simulink model "pattern_separation"  (R2019b)
settings: Solver=FixedStepAuto  StartTime=1  StopTime=simulationtime  FixedStep=stepsize  RelTol=1e-3
values from neighbouring files (symbols this model uses):
  a1 = 0.02    [simulation.m]
  a2 = 0.02    [simulation.m]
  b1 = 0.025    [simulation.m]
  b2 = 0.04    [simulation.m]
  c1 = -65    [simulation.m]
  C1 = normrnd(100,10,[1,nrofgranulecells])    [simulation.m]
  c2 = -65    [simulation.m]
  C2 = normrnd(100,10,[1,nrofinterneurons])    [simulation.m]
  d1 = 6    [simulation.m]
  d2 = 2    [simulation.m]
  inputset = inputsets{no_input}    [simulation.m]
  k1 = 0.25    [simulation.m]
  k2 = 0.25    [simulation.m]
  minimum_saturation_limit_1 = -80    [simulation.m]
  minimum_saturation_limit_2 = -100    [simulation.m]
  noumberofevents = 500    [simulation.m]
  Re = 230    [simulation.m]
  simulationtime = 2000    [simulation.m]
  stepsize = 1    [simulation.m]
  ve1 = -5    [simulation.m]
  ve2 = -80    [simulation.m]
  vr1 = -60    [simulation.m]
  vr2 = -65    [simulation.m]
  vt1 = -55    [simulation.m]
  vt2 = -48    [simulation.m]
undefined symbols (not defined in the file or in its folder): conductancemaxima1, conductancemaxima2, conductancemaxima3, decaytimes1, decaytimes2, decaytimes3, DiscIntNeverNeededParam, Nd, trace
(part 5 of 5)

== matlab function pattern_separation/granule cell 13/MATLAB Function1 ==
  data: eventnoumber input; decaytime output; decaytimes1 input; conductancemaxima1 input; conductancemaximum output
function [decaytime, conductancemaximum] = fcn(eventnoumber, decaytimes1, conductancemaxima1)
if eventnoumber ==0
decaytime =1;
conductancemaximum =0;
else
decaytime = decaytimes1(13, eventnoumber);
conductancemaximum = conductancemaxima1(13, eventnoumber);
end

== matlab function pattern_separation/granule cell 13/MATLAB Function2 ==
  data: eventnoumber input; decaytime output; decaytimes2 input; conductancemaxima2 input; conductancemaximum output
function [decaytime, conductancemaximum] = fcn(eventnoumber, decaytimes2, conductancemaxima2)
if eventnoumber ==0
decaytime =1;
conductancemaximum =0;
else
decaytime = decaytimes2(13, eventnoumber);
conductancemaximum = conductancemaxima2(13, eventnoumber);
end

== matlab function pattern_separation/granule cell 13/granule cell/reset function ==
  data: v input; c input; d input; u input; v1 output; u1 output; r output

function [v1,u1,r] = fcn(v,c,d,u)

if v >= 30
v1= c;
u1 = u+d;
r=1;
else
v1=v;
u1=u;
r=0;  
end

== matlab function pattern_separation/granule cell 1/MATLAB Function2 ==
  data: eventnoumber input; decaytime output; decaytimes2 input; conductancemaxima2 input; conductancemaximum output
function [decaytime, conductancemaximum] = fcn(eventnoumber, decaytimes2, conductancemaxima2)
if eventnoumber ==0
decaytime =1;
conductancemaximum =0;
else
decaytime = decaytimes2(1, eventnoumber);
conductancemaximum = conductancemaxima2(1, eventnoumber);
end

== matlab function pattern_separation/granule cell 1/single exp IPSCs generator (ihibitory synapse)/MATLAB Function ==
  data: inp input; exponential output
function exponential = fcn(inp)

exponential = exp(-inp);

== matlab function pattern_separation/granule cell 13/single exp EPSCs generator (recurrent synapse)/MATLAB Function ==
  data: inp input; exponential output
function exponential = fcn(inp)

exponential = exp(-inp);

== matlab function pattern_separation/granule cell 13/single exp IPSCs generator (ihibitory synapse)/MATLAB Function ==
  data: inp input; exponential output
function exponential = fcn(inp)

exponential = exp(-inp);

== matlab function pattern_separation/granule cell 14/GC neuron/reset function ==
  data: v input; c input; d input; u input; v1 output; u1 output; r output

function [v1,u1,r] = fcn(v,c,d,u)

if v >= 30
v1= c;
u1 = u+d;
r=1;
else
v1=v;
u1=u;
r=0;  
end

== matlab function pattern_separation/granule cell 14/MATLAB Function1 ==
  data: eventnoumber input; decaytime output; decaytimes1 input; conductancemaxima1 input; conductancemaximum output
function [decaytime, conductancemaximum] = fcn(eventnoumber, decaytimes1, conductancemaxima1)
if eventnoumber ==0
decaytime =1;
conductancemaximum =0;
else
decaytime = decaytimes1(14, eventnoumber);
conductancemaximum = conductancemaxima1(14, eventnoumber);
end

== matlab function pattern_separation/granule cell 1/MATLAB Function1 ==
  data: eventnoumber input; decaytime output; decaytimes1 input; conductancemaxima1 input; conductancemaximum output
function [decaytime, conductancemaximum] = fcn(eventnoumber, decaytimes1, conductancemaxima1)
if eventnoumber ==0
decaytime =1;
conductancemaximum =0;
else
decaytime = decaytimes1(1, eventnoumber);
conductancemaximum = conductancemaxima1(1, eventnoumber);
end

== matlab function pattern_separation/granule cell 1/single exp EPSCs generator (recurrent synapse)/MATLAB Function ==
  data: inp input; exponential output
function exponential = fcn(inp)

exponential = exp(-inp);

== matlab function pattern_separation/granule cell 14/MATLAB Function2 ==
  data: eventnoumber input; decaytime output; decaytimes2 input; conductancemaxima2 input; conductancemaximum output
function [decaytime, conductancemaximum] = fcn(eventnoumber, decaytimes2, conductancemaxima2)
if eventnoumber ==0
decaytime =1;
conductancemaximum =0;
else
decaytime = decaytimes2(14, eventnoumber);
conductancemaximum = conductancemaxima2(14, eventnoumber);
end

== matlab function pattern_separation/granule cell 14/single exp EPSCs generator (recurrent synapse)/MATLAB Function ==
  data: inp input; exponential output
function exponential = fcn(inp)

exponential = exp(-inp);

== matlab function pattern_separation/granule cell 14/single exp IPSCs generator (ihibitory synapse)/MATLAB Function ==
  data: inp input; exponential output
function exponential = fcn(inp)

exponential = exp(-inp);

== matlab function pattern_separation/granule cell 15/MATLAB Function1 ==
  data: eventnoumber input; decaytime output; decaytimes1 input; conductancemaxima1 input; conductancemaximum output
function [decaytime, conductancemaximum] = fcn(eventnoumber, decaytimes1, conductancemaxima1)
if eventnoumber ==0
decaytime =1;
conductancemaximum =0;
else
decaytime = decaytimes1(15, eventnoumber);
conductancemaximum = conductancemaxima1(15, eventnoumber);
end

== matlab function pattern_separation/granule cell 15/MATLAB Function2 ==
  data: eventnoumber input; decaytime output; decaytimes2 input; conductancemaxima2 input; conductancemaximum output
function [decaytime, conductancemaximum] = fcn(eventnoumber, decaytimes2, conductancemaxima2)
if eventnoumber ==0
decaytime =1;
conductancemaximum =0;
else
decaytime = decaytimes2(15, eventnoumber);
conductancemaximum = conductancemaxima2(15, eventnoumber);
end

== matlab function pattern_separation/granule cell 15/granule cell/reset function ==
  data: v input; c input; d input; u input; v1 output; u1 output; r output

function [v1,u1,r] = fcn(v,c,d,u)

if v >= 30
v1= c;
u1 = u+d;
r=1;
else
v1=v;
u1=u;
r=0;  
end

== matlab function pattern_separation/granule cell 15/single exp EPSCs generator (recurrent synapse)/MATLAB Function ==
  data: inp input; exponential output
function exponential = fcn(inp)

exponential = exp(-inp);

== matlab function pattern_separation/granule cell 15/single exp IPSCs generator (ihibitory synapse)/MATLAB Function ==
  data: inp input; exponential output
function exponential = fcn(inp)

exponential = exp(-inp);

== matlab function pattern_separation/granule cell 16/GC neuron/reset function ==
  data: v input; c input; d input; u input; v1 output; u1 output; r output

function [v1,u1,r] = fcn(v,c,d,u)

if v >= 30
v1= c;
u1 = u+d;
r=1;
else
v1=v;
u1=u;
r=0;  
end

== matlab function pattern_separation/granule cell 16/MATLAB Function1 ==
  data: eventnoumber input; decaytime output; decaytimes1 input; conductancemaxima1 input; conductancemaximum output
function [decaytime, conductancemaximum] = fcn(eventnoumber, decaytimes1, conductancemaxima1)
if eventnoumber ==0
decaytime =1;
conductancemaximum =0;
else
decaytime = decaytimes1(16, eventnoumber);
conductancemaximum = conductancemaxima1(16, eventnoumber);
end

== matlab function pattern_separation/granule cell 16/MATLAB Function2 ==
  data: eventnoumber input; decaytime output; decaytimes2 input; conductancemaxima2 input; conductancemaximum output
function [decaytime, conductancemaximum] = fcn(eventnoumber, decaytimes2, conductancemaxima2)
if eventnoumber ==0
decaytime =1;
conductancemaximum =0;
else
decaytime = decaytimes2(16, eventnoumber);
conductancemaximum = conductancemaxima2(16, eventnoumber);
end

== matlab function pattern_separation/granule cell 16/single exp EPSCs generator (recurrent synapse)/MATLAB Function ==
  data: inp input; exponential output
function exponential = fcn(inp)

exponential = exp(-inp);

== matlab function pattern_separation/granule cell 16/single exp IPSCs generator (ihibitory synapse)/MATLAB Function ==
  data: inp input; exponential output
function exponential = fcn(inp)

exponential = exp(-inp);

== matlab function pattern_separation/granule cell 9/MATLAB Function1 ==
  data: eventnoumber input; decaytime output; decaytimes1 input; conductancemaxima1 input; conductancemaximum output
function [decaytime, conductancemaximum] = fcn(eventnoumber, decaytimes1, conductancemaxima1)
if eventnoumber ==0
decaytime =1;
conductancemaximum =0;
else
decaytime = decaytimes1(9, eventnoumber);
conductancemaximum = conductancemaxima1(9, eventnoumber);
end

== matlab function pattern_separation/granule cell 9/MATLAB Function2 ==
  data: eventnoumber input; decaytime output; decaytimes2 input; conductancemaxima2 input; conductancemaximum output
function [decaytime, conductancemaximum] = fcn(eventnoumber, decaytimes2, conductancemaxima2)
if eventnoumber ==0
decaytime =1;
conductancemaximum =0;
else
decaytime = decaytimes2(9, eventnoumber);
conductancemaximum = conductancemaxima2(9, eventnoumber);
end

== matlab function pattern_separation/granule cell 9/granule cell/reset function ==
  data: v input; c input; d input; u input; v1 output; u1 output; r output

function [v1,u1,r] = fcn(v,c,d,u)

if v >= 30
v1= c;
u1 = u+d;
r=1;
else
v1=v;
u1=u;
r=0;  
end

== matlab function pattern_separation/granule cell 9/single exp EPSCs generator (recurrent synapse)/MATLAB Function ==
  data: inp input; exponential output
function exponential = fcn(inp)

exponential = exp(-inp);

== matlab function pattern_separation/granule cell 9/single exp IPSCs generator (ihibitory synapse)/MATLAB Function ==
  data: inp input; exponential output
function exponential = fcn(inp)

exponential = exp(-inp);

== matlab function pattern_separation/stimulation (pattern generator)/MATLAB Function ==
  data: iteration input; integrator input; trigger output; spiketrains input
function trigger = fcn(iteration, integrator,spiketrains)
trigger = spiketrains(iteration,integrator);

== matlab function pattern_separation/granule cell 17/MATLAB Function1 ==
  data: eventnoumber input; decaytime output; decaytimes1 input; conductancemaxima1 input; conductancemaximum output
function [decaytime, conductancemaximum] = fcn(eventnoumber, decaytimes1, conductancemaxima1)
if eventnoumber ==0
decaytime =1;
conductancemaximum =0;
else
decaytime = decaytimes1(17, eventnoumber);
conductancemaximum = conductancemaxima1(17, eventnoumber);
end

== matlab function pattern_separation/granule cell 17/MATLAB Function2 ==
  data: eventnoumber input; decaytime output; decaytimes2 input; conductancemaxima2 input; conductancemaximum output
function [decaytime, conductancemaximum] = fcn(eventnoumber, decaytimes2, conductancemaxima2)
if eventnoumber ==0
decaytime =1;
conductancemaximum =0;
else
decaytime = decaytimes2(17, eventnoumber);
conductancemaximum = conductancemaxima2(17, eventnoumber);
end

== matlab function pattern_separation/granule cell 17/granule cell/reset function ==
  data: v input; c input; d input; u input; v1 output; u1 output; r output

function [v1,u1,r] = fcn(v,c,d,u)

if v >= 30
v1= c;
u1 = u+d;
r=1;
else
v1=v;
u1=u;
r=0;  
end

== matlab function pattern_separation/granule cell 17/single exp EPSCs generator (recurrent synapse)/MATLAB Function ==
  data: inp input; exponential output
function exponential = fcn(inp)

exponential = exp(-inp);

== matlab function pattern_separation/granule cell 17/single exp IPSCs generator (ihibitory synapse)/MATLAB Function ==
  data: inp input; exponential output
function exponential = fcn(inp)

exponential = exp(-inp);

== matlab function pattern_separation/granule cell 18/GC neuron/reset function ==
  data: v input; c input; d input; u input; v1 output; u1 output; r output

function [v1,u1,r] = fcn(v,c,d,u)

if v >= 30
v1= c;
u1 = u+d;
r=1;
else
v1=v;
u1=u;
r=0;  
end

== matlab function pattern_separation/granule cell 18/MATLAB Function1 ==
  data: eventnoumber input; decaytime output; decaytimes1 input; conductancemaxima1 input; conductancemaximum output
function [decaytime, conductancemaximum] = fcn(eventnoumber, decaytimes1, conductancemaxima1)
if eventnoumber ==0
decaytime =1;
conductancemaximum =0;
else
decaytime = decaytimes1(18, eventnoumber);
conductancemaximum = conductancemaxima1(18, eventnoumber);
end

== matlab function pattern_separation/granule cell 18/MATLAB Function2 ==
  data: eventnoumber input; decaytime output; decaytimes2 input; conductancemaxima2 input; conductancemaximum output
function [decaytime, conductancemaximum] = fcn(eventnoumber, decaytimes2, conductancemaxima2)
if eventnoumber ==0
decaytime =1;
conductancemaximum =0;
else
decaytime = decaytimes2(18, eventnoumber);
conductancemaximum = conductancemaxima2(18, eventnoumber);
end

== matlab function pattern_separation/granule cell 18/single exp EPSCs generator (recurrent synapse)/MATLAB Function ==
  data: inp input; exponential output
function exponential = fcn(inp)

exponential = exp(-inp);

== matlab function pattern_separation/granule cell 18/single exp IPSCs generator (ihibitory synapse)/MATLAB Function ==
  data: inp input; exponential output
function exponential = fcn(inp)

exponential = exp(-inp);

== matlab function pattern_separation/granule cell 19/MATLAB Function1 ==
  data: eventnoumber input; decaytime output; decaytimes1 input; conductancemaxima1 input; conductancemaximum output
function [decaytime, conductancemaximum] = fcn(eventnoumber, decaytimes1, conductancemaxima1)
if eventnoumber ==0
decaytime =1;
conductancemaximum =0;
else
decaytime = decaytimes1(19, eventnoumber);
conductancemaximum = conductancemaxima1(19, eventnoumber);
end

== matlab function pattern_separation/granule cell 19/MATLAB Function2 ==
  data: eventnoumber input; decaytime output; decaytimes2 input; conductancemaxima2 input; conductancemaximum output
function [decaytime, conductancemaximum] = fcn(eventnoumber, decaytimes2, conductancemaxima2)
if eventnoumber ==0
decaytime =1;
conductancemaximum =0;
else
decaytime = decaytimes2(19, eventnoumber);
conductancemaximum = conductancemaxima2(19, eventnoumber);
end

== matlab function pattern_separation/granule cell 19/granule cell/reset function ==
  data: v input; c input; d input; u input; v1 output; u1 output; r output

function [v1,u1,r] = fcn(v,c,d,u)

if v >= 30
v1= c;
u1 = u+d;
r=1;
else
v1=v;
u1=u;
r=0;  
end

== matlab function pattern_separation/granule cell 19/single exp EPSCs generator (recurrent synapse)/MATLAB Function ==
  data: inp input; exponential output
function exponential = fcn(inp)

exponential = exp(-inp);

== matlab function pattern_separation/granule cell 19/single exp IPSCs generator (ihibitory synapse)/MATLAB Function ==
  data: inp input; exponential output
function exponential = fcn(inp)

exponential = exp(-inp);

== matlab function pattern_separation/granule cell 20/GC neuron/reset function ==
  data: v input; c input; d input; u input; v1 output; u1 output; r output

function [v1,u1,r] = fcn(v,c,d,u)

if v >= 30
v1= c;
u1 = u+d;
r=1;
else
v1=v;
u1=u;
r=0;  
end

== matlab function pattern_separation/granule cell 20/MATLAB Function1 ==
  data: eventnoumber input; decaytime output; decaytimes1 input; conductancemaxima1 input; conductancemaximum output
function [decaytime, conductancemaximum] = fcn(eventnoumber, decaytimes1, conductancemaxima1)
if eventnoumber ==0
decaytime =1;
conductancemaximum =0;
else
decaytime = decaytimes1(20, eventnoumber);
conductancemaximum = conductancemaxima1(20, eventnoumber);
end

== matlab function pattern_separation/granule cell 20/MATLAB Function2 ==
  data: eventnoumber input; decaytime output; decaytimes2 input; conductancemaxima2 input; conductancemaximum output
function [decaytime, conductancemaximum] = fcn(eventnoumber, decaytimes2, conductancemaxima2)
if eventnoumber ==0
decaytime =1;
conductancemaximum =0;
else
decaytime = decaytimes2(1, eventnoumber);
conductancemaximum = conductancemaxima2(1, eventnoumber);
end

== matlab function pattern_separation/granule cell 20/single exp EPSCs generator (recurrent synapse)/MATLAB Function ==
  data: inp input; exponential output
function exponential = fcn(inp)

exponential = exp(-inp);

== matlab function pattern_separation/granule cell 20/single exp IPSCs generator (ihibitory synapse)/MATLAB Function ==
  data: inp input; exponential output
function exponential = fcn(inp)

exponential = exp(-inp);

== matlab function pattern_separation/LFP/MATLAB Function ==
  data: GC_cell_1_current input; GC_cell_2_current input; GC_cell_3_current input; GC_cell_4_current input; GC_cell_5_current input; GC_cell_6_current input; GC_cell_7_current input; GC_cell_8_current input; GC_cell_9_current input; GC_cell_10_current input; GC_cell_11_current input; GC_cell_12_current input; GC_cell_13_current input; GC_cell_14_current input; GC_cell_15_current input; GC_cell_16_current input; GC_cell_17_current input; GC_cell_18_current input; GC_cell_19_current input; GC_cell_20_current input; interneuron_1_current input; interneuron_2_current input; extracellural_current output; Nd input
function extracellural_current = fcn(...
    GC_cell_1_current,...
    GC_cell_2_current,...
    GC_cell_3_current,...
    GC_cell_4_current,...
    GC_cell_5_current,...
    GC_cell_6_current,...
    GC_cell_7_current,...
    GC_cell_8_current,...
    GC_cell_9_current,...
    GC_cell_10_current,...
    GC_cell_11_current,...
    GC_cell_12_current,...
    GC_cell_13_current,...
    GC_cell_14_current,...
    GC_cell_15_current,...
    GC_cell_16_current,...
    GC_cell_17_current,...
    GC_cell_18_current,...
    GC_cell_19_current,...
    GC_cell_20_current,...
    interneuron_1_current,...
    interneuron_2_current,...
    Nd)

extracellural_current =...
    GC_cell_1_current/Nd(1)+...
    GC_cell_2_current/Nd(2)+...
    GC_cell_3_current/Nd(3)+...
    GC_cell_4_current/Nd(4)+...
    GC_cell_5_current/Nd(5)+...
    GC_cell_6_current/Nd(6)+...
    GC_cell_7_current/Nd(7)+...
    GC_cell_8_current/Nd(8)+...
    GC_cell_9_current/Nd(9)+...
    GC_cell_10_current/Nd(10)+...
    GC_cell_11_current/Nd(11)+...
    GC_cell_12_current/Nd(12)+...
    GC_cell_13_current/Nd(13)+...
    GC_cell_14_current/Nd(14)+...
    GC_cell_15_current/Nd(15)+...
    GC_cell_16_current/Nd(16)+...
    GC_cell_17_current/Nd(17)+...
    GC_cell_18_current/Nd(18)+...
    GC_cell_19_current/Nd(19)+...
    GC_cell_20_current/Nd(20)+...
    interneuron_1_current/Nd(21)+...
    interneuron_2_current/Nd(22);
